simulink model "UAV_translational_dynamics"  (R2016a)
settings: Solver=VariableStepAuto  StartTime=0.0  StopTime=10.0  RelTol=1e-3
values from neighbouring files (symbols this model uses):
  g = 9.81    [init_UAV_model.m]
  m = 29e-3    (= 0.029)    [init_UAV_model.m]
  p0 = [0;0;0]    [init_UAV_model.m]
  v0 = [0;0;0]    [init_UAV_model.m]
settings Model: Creator=mgreiff  LastModifiedBy=mgreiff

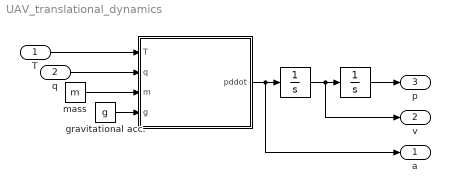
== system UAV_translational_dynamics ==
  T : Inport  PortDimensions=1
  q : Inport  Port=2  PortDimensions=4
  " " : MATLAB Function  TreatAsAtomicUnit=on
  "    " : Integrator  InitialCondition=v0
  "      " : Integrator  InitialCondition=p0
  gravitational acc. : Constant  Value=g
  mass : Constant  Value=m
  a : Outport  PortDimensions=3
  v : Outport  Port=2  PortDimensions=3
  p : Outport  Port=3  PortDimensions=3
  wires:
  " "/1(pddot) -> a/1, "    "/1
  mass/1 -> " "/3(m)
  q/1 -> " "/2(q)
  T/1 -> " "/1(T)
  "    "/1 -> v/1, "      "/1
  "      "/1 -> p/1
  gravitational acc./1 -> " "/4(g)

== matlab function UAV_translational_dynamics/  ==
  data: T input; q input; m input; pddot output; g input
function pddot  = f(T, q, m, g)
% ~~~ Copyright (c) 2018 Marcus Greiff (see LICENCE.md) ~~~
%
% Model of the translational dynamics, a subset of the UAV dynamics
%
%    pddot  = f(T, q, m, g)
%
% The inputs to this subsystem are is the total thrust generated by the
% rotors, T, as well as a quaternion attitude (which is not assumed to be
% normalized). The equations are parametrized by the graviational constant,
% g, and the UAV mass, m.

q = q./norm(q);
qThrust = [0;0;0;T];
qTemp    = leftProduct(q) * qThrust;
qRotated = leftProduct(qTemp) * inverse(q);
pddot = (1/m).*imaginary(qRotated) - [0;0;g];
end


function S = skew(v)
    vx = v(1);
    vy = v(2);
    vz = v(3);
    S = [0 -vz vy; vz 0 -vx; -vy vx 0];
end

function qL = leftProduct(q)
    qw = q(1);
    qv = q(2:4);
    qL = qw*eye(4) + [0, -qv'; qv, skew(qv)];
end

function qinv = inverse(q)
    qinv=zeros(4,1);
    qinv(1) = q(1);
    qinv(2:4) = -q(2:4);
end

function qreal = real(q)
    qreal = q(1);
end

function qimaginary = imaginary(q)
    qimaginary = q(2:4);
end

function value = sign(v)
    if v >= 0
        value = 1;
    elseif v < 0
        value = -1;
    else
        value = 0;
    end
end
